simulink model "attitudePropagate"  (R2023b)
settings: Solver=VariableStepAuto  StartTime=0.0  StopTime=Tfinal  RelTol=1e-3
settings Model: Creator=stanforduser  LastModifiedBy=stanforduser

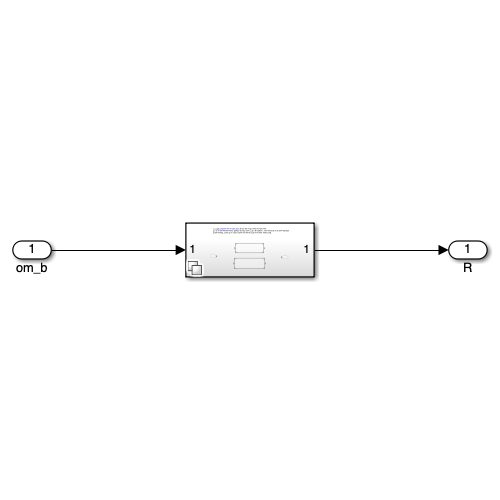
[thumbnail: Simulink's stored preview of the top-level diagram]
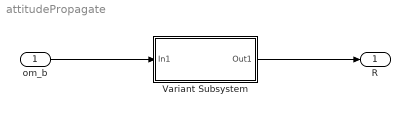
== system attitudePropagate ==
  om_b : Inport
  Variant Subsystem : Subsystem  Variant=on
  R : Outport
  wires:
  om_b/1 -> Variant Subsystem/1(In1)
  Variant Subsystem/1(Out1) -> R/1

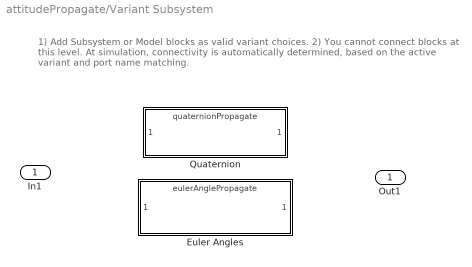
== system attitudePropagate/Variant Subsystem ==
  note: 1) Add Subsystem or Model blocks as valid variant choices.
      | 2) You cannot connect blocks at this level. At simulation, connectivity is automatically
      | determined, based on the active variant and port name matching.
  In1 : Inport
  Euler Angles : ModelReference  ModelNameDialog=eulerAnglePropagate.slx  SimulationMode=Normal  VariantControl=Type==1  ModelReferenceVersion=1.3
  Quaternion : ModelReference  ModelNameDialog=quaternionPropagate.slx  SimulationMode=Normal  VariantControl=Type==2  ModelReferenceVersion=1.3
  Out1 : Outport
